simulink model "model_silnik_dykretny_lock"  (R2020b)
settings: Solver=FixedStepDiscrete  StartTime=0.0  StopTime=stopTime  FixedStep=h  RelTol=1e-3
values from neighbouring files (symbols this model uses):
  u_0 = 1    [start_model_silnik.m]    (also in staticChar.mat = -2)
settings Model: Creator=Rafal  LastModifiedBy=Robert
settings DataIOCC: ReturnWorkspaceOutputs=off

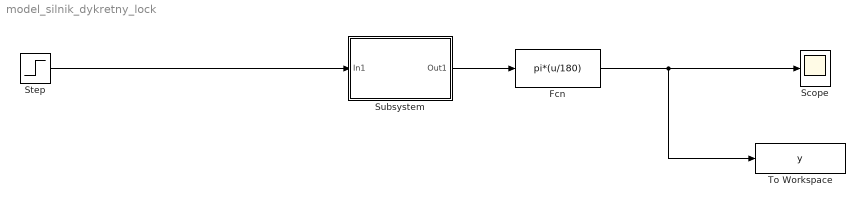
== system model_silnik_dykretny_lock ==
  Fcn : Fcn  Expr=pi*(u/180)
  Scope : Scope
  Step : Step  Time=0  After=u_0  SampleTime=0
  Subsystem : Subsystem
  To Workspace : ToWorkspace  VariableName=y  SaveFormat=Timeseries  SampleTime=-1
  wires:
  Step/1 -> Subsystem/1(In1)
  Subsystem/1(Out1) -> Fcn/1
  Fcn/1 -> To Workspace/1, Scope/1

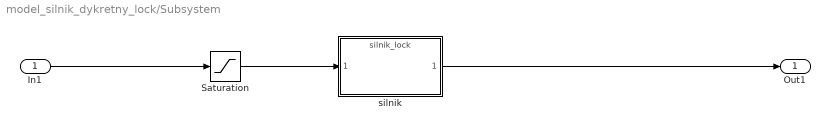
== system model_silnik_dykretny_lock/Subsystem ==
  In1 : Inport
  Saturation : Saturate  UpperLimit=2  LowerLimit=-2
  silnik : ModelReference  ModelNameDialog=silnik_lock.slxp  ModelReferenceVersion=1.38  CopyOfModelProtected=on
  Out1 : Outport
  wires:
  silnik/1 -> Out1/1
  Saturation/1 -> silnik/1
  In1/1 -> Saturation/1
